simulink library "libMdl_Gnss"  (R2018a)
settings: Solver=VariableStepAuto  StartTime=0.0  StopTime=10.0  RelTol=1e-3
libraries: dspsrcs4 x1
settings Model: Creator=hwinter  LastModifiedBy=hwinter

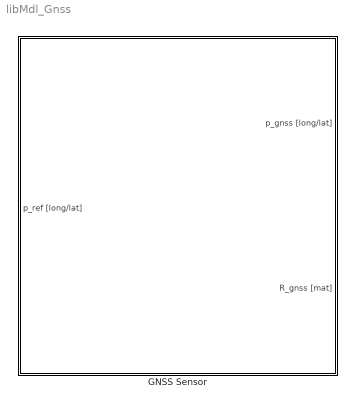
== system libMdl_Gnss ==
  GNSS Sensor : Subsystem  TreatAsAtomicUnit=on  SystemSampleTime=mv_T_gnss  mask(GNSS Sensor){mv_T_gnss=-1, mv_sigma_gnss=[], mv_z_0_gnss=[], mv_seed_gnss=[]}
      mask prompts: mv_T_gnss "Sample time:"; mv_sigma_gnss "sigma_w:"; mv_z_0_gnss "z_0:"; mv_seed_gnss "Seed:"
      mask help:
      | Sample Time:
      | Sample time of the block in seconds
      |
      | sigma_w:
      | Standard deviation of the position output
      | (format: [sigma_longitude, sigma_latitude])
      |
      | z_0:
      | Initial position
      | (format: [p_0_longitude, p_0_latitude])
      |
      | Seed:
      | Choose the behaviour of the random generator
      mask init:
      | % parameter_field_name = 'RepMode';
      | % type_options = {'Repeatable','Not repeatable'};
      | % 
      | % block_handle = find_system(gcbh,'LookUnderMasks','all','Name','rnd_src');
      | % set_param(block_handle,parameter_field_name,type_options{mv_rep_mode});
      mask Display:
      | str1 = sprintf('\\color{black}{\\bf GNSS}\n\n');
      | str2 = sprintf('Sample Time: %0.2f\n\n',mv_T_gnss);
      | if length(mv_sigma_gnss) > 1
      |     str3 = sprintf('\\sigma_{long}: %0.2f\n',mv_sigma_gnss(1));
      |     str4 = sprintf('\\sigma_{lat}: %0.2f\n',mv_sigma_gnss(2));
      | else
      |     str3 = sprintf('\\sigma_{long}: []\n');
      |     str4 = sprintf('\\sigma_{lat}: []\n');
      | 
      | end % if
      | if length(mv_z_0_gnss) <= 3
      |     str5 = sprintf('z_0: %s\n\n',mat2str(mv_z_0_gnss,5));
      | else
      |     str5 = sprintf('z_0: [...]\n\n');
      | end % if
      | 
      | str6 = sprintf('Seed: %i\n\n',mv_seed_gnss);
      | 
      | 
      | str = [str1,str2,str3,str4,str5,str6];
      | 
      | text( 0.5,0.5, ...
      |       str, ...
      |       'horizontalAlignment', 'center', ...
      |       'texmode','on' ...
      |     )

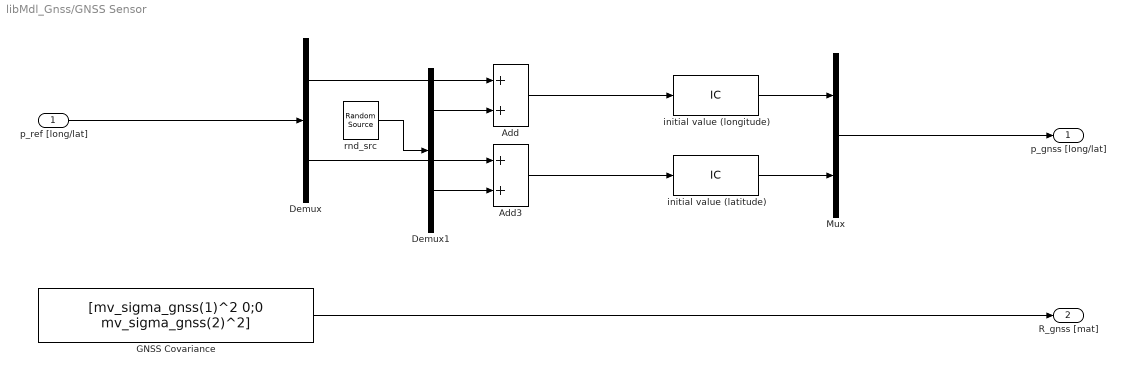
== system libMdl_Gnss/GNSS Sensor ==
  p_ref [long/lat] : Inport
  Add : Sum
  Add3 : Sum
  Demux : Demux  Outputs=2
  Demux1 : Demux  Outputs=2
  GNSS Covariance : Constant  Value=[mv_sigma_gnss(1)^2 0;0 mv_sigma_gnss(2)^2]
  Mux : Mux  Inputs=2
  initial value (latitude) : InitialCondition  Value=mv_z_0_gnss(2)
  initial value (longitude) : InitialCondition  Value=mv_z_0_gnss(1)
  rnd_src : dspsrcs4/Random Source  SrcType=Gaussian  NormMethod=Ziggurat  CltLength=12  MinVal=0  MaxVal=1  MeanVal=[0 0]  VarVal=mv_sigma_gnss.^2  RepMode=Specify seed  rawSeed=mv_seed_gnss  IsInherit=on  SampMode=Discrete  SampTime=1  SampFrame=1  DataType=Double  OutComplex=Real  OutputFrames=off
  p_gnss [long/lat] : Outport
  R_gnss [mat] : Outport  Port=2
  wires:
  initial value (latitude)/1 -> Mux/2
  initial value (longitude)/1 -> Mux/1
  Mux/1 -> p_gnss [long/lat]/1
  GNSS Covariance/1 -> R_gnss [mat]/1
  p_ref [long/lat]/1 -> Demux/1
  Demux/1 -> Add/1
  Demux/2 -> Add3/1
  Add/1 -> initial value (longitude)/1
  Add3/1 -> initial value (latitude)/1
  Demux1/1 -> Add/2
  Demux1/2 -> Add3/2
  rnd_src/1 -> Demux1/1
